simulink model "aero_guidance"  (R2019b)
settings: Solver=ode45  StartTime=0.0  StopTime=20  RelTol=1e-3  AbsTol=1e-6
PreLoadFcn:
  | aero_guid_dat
StopFcn:
  | aero_guid_plot
undefined symbols (not defined in the file): Beamwidth, Cm_el, Cm_q, Cz_el, d2r, d_ref, fin_max, fin_min, g, h_ini, K_r, Ks, l_acc, max_acc, max_gimbal, min_gimbal, pos_tgt, S_ref, theta_tgt, Thrust, tors, v_tgt, wgyro, wn_hom, x_ini
libraries: simulink_need_slupdate x11, aerospace x5, simulink x1
CloseFcn:
  | h=findobj('type','figure');if ~isempty(h);close(h);end
Description:
  | Dynamics of a missile engaging a target which is flying straight and level
settings Model: ExtModeTrigMode=oneshot  ExtModeArmWhenConnect=off  ExtModeAutoUpdateStatusClock=off  Creator=The MathWorks, Inc.  LastModifiedBy=Eduardo
settings SolverCC: AutoScaleAbsTol=off
settings DataIOCC: SaveFormat=Array  SaveOutput=off  ReturnWorkspaceOutputs=off  StateSaveName=xbase  OutputSaveName=ybase  SignalLoggingName=sigsOut
settings OptimizationCC: BlockReduction=off  ExpressionDepthLimit=2147483647  InitFltsAndDblsToZero=on  LifeSpan=inf
settings DebuggingCC: SaveWithParameterizedLinksMsg=none  SignalResolutionControl=TryResolveAllWithWarning  MultiTaskDSMMsg=warning  MultiTaskCondExecSysMsg=none  SigSpecEnsureSampleTimeMsg=none  FcnCallInpInsideContextMsg=warning  StateNameClashWarn=warning  SFUnexpectedBacktrackingDiag=warning  SFNoUnconditionalDefaultTransitionDiag=warning  SFExecutionAtInitializationDiag=none  ArithmeticOperatorsInVariantConditions=warning
settings HardwareCC: ProdBitPerPointer=32  ProdBitPerSizeT=32  ProdBitPerPtrDiffT=32  ProdLargestAtomicFloat=None  ProdIntDivRoundTo=Undefined  ProdEndianess=Unspecified  ProdWordSize=32  ProdHWDeviceType=32-bit Generic
settings ModelReferenceCC: PropagateSignalLabelsOutOfModel=off
settings SFSimCC: SimUseLocalCustomCode=off  SimParseCustomCode=off  CustomCodeUndefinedFunction=UseInterfaceOnly
settings RTWCC: RTWUseLocalCustomCode=off
settings CodeAppCC: StateflowObjectComments=on
settings GRTTargetCC: TargetFcnLib=ansi_tfl_tmw.mat  TargetLangStandard=C89/C90 (ANSI)  GeneratePreprocessorConditionals=Disable all  CombineOutputUpdateFcns=off  GRTInterface=on
settings ConfigComp: CovMetricSettings=d  CovHtmlReporting=on  CovSaveCumulativeToWorkspaceVar=on  CovSaveSingleToWorkspaceVar=on  CovExternalEMLEnable=off  CovSFcnEnable=off

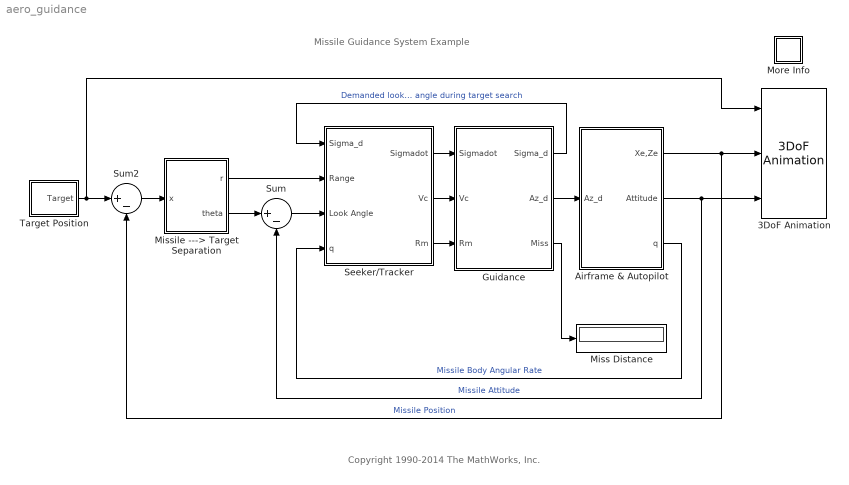
== system aero_guidance ==
  note: Copyright 1990-2014 The MathWorks, Inc.
  note: Missile Guidance System Example
  3DoF Animation : aerospace/Animation/3DoF Animation  u1=[0 5000 -2000 2000 -5050 -3050]  u2=0.03  u3=1.8  u5=Fly alongside  u6=[200 200 -50]  u7=20  u8=on
  Airframe & Autopilot : Subsystem
  Guidance : Subsystem
  Miss Distance : Display
  Missile ---> Target Separation : Subsystem  mask(Cart2Polar){}
      mask help:
      | Transformation from cartesian to polar coordinates.
      | [x, y] -> [r, theta]
      |
      | r = sqrt(x^2 + y^2);
      | theta = atan(y/x);
      mask Help: Unmask this block for more help.
      mask Display: plot(0,0,100,100,[24,20,15,20,20],[85,95,85,95,20],[80,20,95,85,95,85],[70,20,20,15,20,24],[56,56,55,52,50,46],[20,26,31,35,38,42])
  More Info : Subsystem
      settings: OpenFcn=showdemo(bdroot(gcb))
      mask Display: disp('?')
  Seeker/Tracker : Subsystem
  Sum : Sum  Inputs=|+-  SaturateOnIntegerOverflow=on  InputSameDT=on  OutDataTypeStr=Inherit: Same as first input
  Sum2 : Sum  Inputs=|+-  SaturateOnIntegerOverflow=on  InputSameDT=on  OutDataTypeStr=Inherit: Same as first input
  Target Position : Subsystem
  wires:
  Missile ---> Target Separation/2(theta) -> Sum/1
  Guidance/2(Az_d) -> Airframe & Autopilot/1(Az_d)
  Seeker/Tracker/2(Vc) -> Guidance/2(Vc)
  Seeker/Tracker/3(Rm) -> Guidance/3(Rm)
  Guidance/3(Miss) -> Miss Distance/1
  Seeker/Tracker/1(Sigmadot) -> Guidance/1(Sigmadot)
  Sum/1 -> Seeker/Tracker/3(Look Angle)
  Airframe & Autopilot/3(q) -> Seeker/Tracker/4(q)  "Missile Body Angular Rate"
  Guidance/1(Sigma_d) -> Seeker/Tracker/1(Sigma_d)  "Demanded look angle during target search"
  Missile ---> Target Separation/1(r) -> Seeker/Tracker/2(Range)
  Airframe & Autopilot/1(Xe,Ze) -> 3DoF Animation/2, Sum2/2  "Missile Position"
  Airframe & Autopilot/2(Attitude) -> 3DoF Animation/3, Sum/2  "Missile Attitude"
  Target Position/1(Target) -> Sum2/1, 3DoF Animation/1
  Sum2/1 -> Missile ---> Target Separation/1(x)

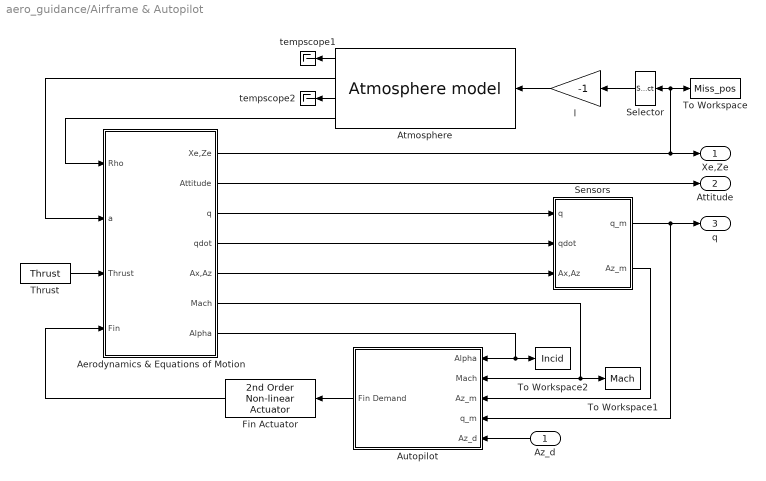
== system aero_guidance/Airframe & Autopilot ==
  Az_d : Inport
  Aerodynamics & Equations of Motion : Subsystem
  Atmosphere : aerospace/Atmosphere/Atmosphere model
  Autopilot : Subsystem
  Fin Actuator : aerospace/Actuators/2nd Order Non-linear Actuator  wn_fin=wn_fin  z_fin=z_fin  fin_max=fin_max  fin_min=fin_min  fin_maxrate=fin_maxrate  fin_act_0=fin_act_0
  Selector : Selector  InputPortWidth=2  IndexOptions=Index vector (dialog)  Indices=[2]  OutputSizes=1
  Sensors : Subsystem
  Thrust : Constant  Value=Thrust
  To Workspace : ToWorkspace  VariableName=Miss_pos  SaveFormat=Structure With Time  SampleTime=-1
  To Workspace1 : ToWorkspace  VariableName=Mach  SaveFormat=Structure With Time  SampleTime=-1
  To Workspace2 : ToWorkspace  VariableName=Incid  SaveFormat=Structure With Time  SampleTime=-1
  l : Gain  Gain=-1  SaturateOnIntegerOverflow=on  OutDataTypeStr=Inherit: Same as input  ParamDataTypeStr=Inherit: Same as input
  tempscope1 : Terminator
  tempscope2 : Terminator
  Xe,Ze : Outport  InitialOutput=0  VectorParamsAs1DForOutWhenUnconnected=off
  Attitude : Outport  Port=2  InitialOutput=0  VectorParamsAs1DForOutWhenUnconnected=off
  q : Outport  Port=3  InitialOutput=0  VectorParamsAs1DForOutWhenUnconnected=off
  wires:
  Aerodynamics & Equations of Motion/2(Attitude) -> Attitude/1
  Thrust/1 -> Aerodynamics & Equations of Motion/3(Thrust)
  Atmosphere/3 -> tempscope2/1
  Atmosphere/4 -> Aerodynamics & Equations of Motion/1(Rho)
  Atmosphere/1 -> tempscope1/1
  Atmosphere/2 -> Aerodynamics & Equations of Motion/2(a)
  Selector/1 -> l/1
  l/1 -> Atmosphere/1
  Aerodynamics & Equations of Motion/5(Ax,Az) -> Sensors/3(Ax,Az)
  Aerodynamics & Equations of Motion/4(qdot) -> Sensors/2(qdot)
  Aerodynamics & Equations of Motion/1(Xe,Ze) -> Xe,Ze/1, To Workspace/1, Selector/1
  Az_d/1 -> Autopilot/5(Az_d)
  Autopilot/1(Fin Demand) -> Fin Actuator/1
  Fin Actuator/1 -> Aerodynamics & Equations of Motion/4(Fin)
  Aerodynamics & Equations of Motion/7(Alpha) -> Autopilot/1(Alpha), To Workspace2/1
  Sensors/2(Az_m) -> Autopilot/3(Az_m)
  Aerodynamics & Equations of Motion/6(Mach) -> Autopilot/2(Mach), To Workspace1/1
  Sensors/1(q_m) -> Autopilot/4(q_m), q/1
  Aerodynamics & Equations of Motion/3(q) -> Sensors/1(q)

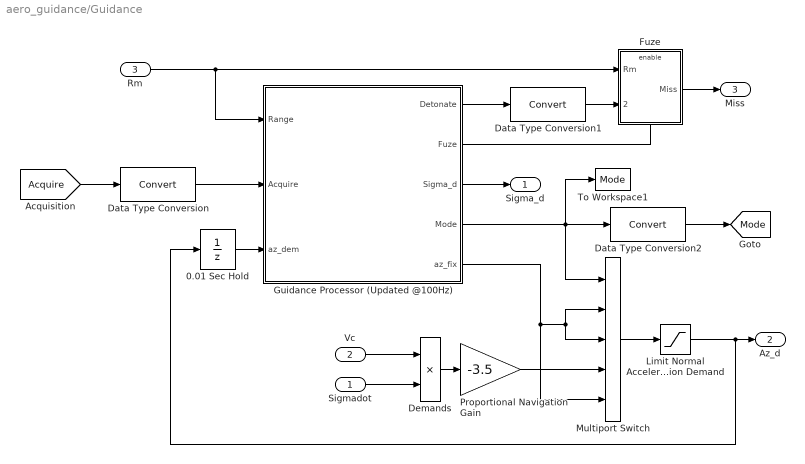
== system aero_guidance/Guidance ==
  Sigmadot : Inport
  Vc : Inport  Port=2
  Rm : Inport  Port=3
  0.01 Sec Hold : UnitDelay  SampleTime=0.01  HasFrameUpgradeWarning=on
  Data Type Conversion : DataTypeConversion
  Data Type Conversion1 : DataTypeConversion
  Data Type Conversion2 : DataTypeConversion
  Demands : Product  SaturateOnIntegerOverflow=on  InputSameDT=on  OutDataTypeStr=Inherit: Same as first input
  Fuze : Subsystem  TreatAsAtomicUnit=on
  Guidance Processor (Updated @100Hz) : Stateflow chart  TreatAsAtomicUnit=on
  "Limit Normal Acceleration Demand " : Saturate  UpperLimit=max_acc  LowerLimit=-max_acc
  Multiport Switch : MultiPortSwitch  Inputs=4  SaturateOnIntegerOverflow=on  InputSameDT=on
  Proportional Navigation Gain : Gain  Gain=-3.5  SaturateOnIntegerOverflow=on  OutDataTypeStr=Inherit: Same as input  ParamDataTypeStr=Inherit: Same as input
  To Workspace1 : ToWorkspace  VariableName=Mode  SaveFormat=Structure With Time
  Sigma_d : Outport  VectorParamsAs1DForOutWhenUnconnected=off
  Az_d : Outport  Port=2  VectorParamsAs1DForOutWhenUnconnected=off
  Miss : Outport  Port=3  VectorParamsAs1DForOutWhenUnconnected=off
  tag scope: Mode=global
  wires:
  Fuze/1("Miss ") -> Miss/1
  Guidance Processor (Updated @100Hz)/3(Sigma_d) -> Sigma_d/1
  [Acquire] -> Data Type Conversion/1
  Multiport Switch/1 -> "Limit Normal Acceleration Demand "/1
  Guidance Processor (Updated @100Hz)/1(Detonate) -> Data Type Conversion1/1
  "Limit Normal Acceleration Demand "/1 -> Az_d/1, 0.01 Sec Hold/1
  Guidance Processor (Updated @100Hz)/5(az_fix) -> Multiport Switch/2, Multiport Switch/3, Multiport Switch/5
  0.01 Sec Hold/1 -> Guidance Processor (Updated @100Hz)/3(az_dem)
  Sigmadot/1 -> Demands/2
  Proportional Navigation Gain/1 -> Multiport Switch/4
  Vc/1 -> Demands/1
  Demands/1 -> Proportional Navigation Gain/1
  Rm/1 -> Fuze/1(Rm), Guidance Processor (Updated @100Hz)/1(Range)
  Guidance Processor (Updated @100Hz)/2(Fuze) -> Fuze/Enable
  Guidance Processor (Updated @100Hz)/4(Mode) -> Data Type Conversion2/1, To Workspace1/1, Multiport Switch/1
  Data Type Conversion/1 -> Guidance Processor (Updated @100Hz)/2(Acquire)
  Data Type Conversion1/1 -> Fuze/2(Detonate)
  Data Type Conversion2/1 -> [Mode]

== system aero_guidance/Missile ---> Target Separation ==
  x : Inport
  Range : Fcn  Expr=hypot(u[1],u[2])
  Sightline Angle : Fcn  Expr=atan2(-u[2],u[1])
  r : Outport  InitialOutput=0  VectorParamsAs1DForOutWhenUnconnected=off
  theta : Outport  Port=2  InitialOutput=0  VectorParamsAs1DForOutWhenUnconnected=off
  wires:
  x/1 -> Sightline Angle/1, Range/1
  Range/1 -> r/1
  Sightline Angle/1 -> theta/1

== system aero_guidance/More Info ==

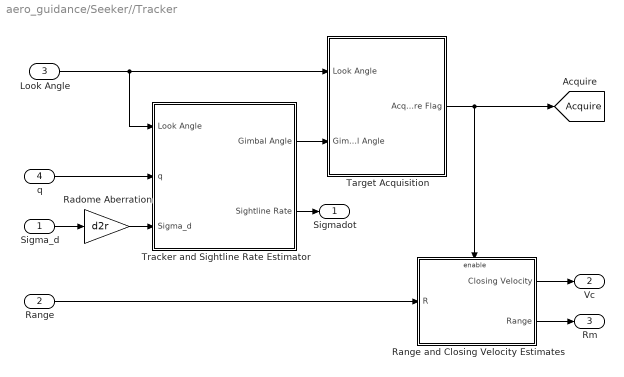
== system aero_guidance/Seeker//Tracker ==
  Sigma_d : Inport
  Range : Inport  Port=2
  Look Angle : Inport  Port=3
  q : Inport  Port=4
  Radome Aberration : Gain  Gain=d2r  SaturateOnIntegerOverflow=on  OutDataTypeStr=Inherit: Same as input  ParamDataTypeStr=Inherit: Same as input
  Range and Closing Velocity Estimates : Subsystem  TreatAsAtomicUnit=on
  Target Acquisition : Subsystem
  Tracker and Sightline Rate Estimator : Subsystem
  Sigmadot : Outport  VectorParamsAs1DForOutWhenUnconnected=off
  Vc : Outport  Port=2  VectorParamsAs1DForOutWhenUnconnected=off
  Rm : Outport  Port=3  VectorParamsAs1DForOutWhenUnconnected=off
  tag scope: Acquire=global
  wires:
  Tracker and Sightline Rate Estimator/2(Sightline Rate) -> Sigmadot/1
  Radome Aberration/1 -> Tracker and Sightline Rate Estimator/3(Sigma_d)
  Tracker and Sightline Rate Estimator/1("Gimbal Angle ") -> Target Acquisition/2(Gimbal Angle)
  Target Acquisition/1(Acquire Flag) -> [Acquire], Range and Closing Velocity Estimates/Enable
  q/1 -> Tracker and Sightline Rate Estimator/2(q)
  Look Angle/1 -> Target Acquisition/1(Look Angle), Tracker and Sightline Rate Estimator/1(Look Angle)
  Range/1 -> Range and Closing Velocity Estimates/1(R)
  Range and Closing Velocity Estimates/2(Range) -> Rm/1
  Range and Closing Velocity Estimates/1(Closing Velocity) -> Vc/1
  Sigma_d/1 -> Radome Aberration/1

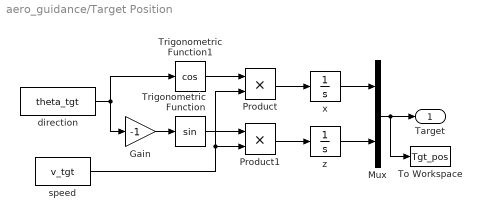
== system aero_guidance/Target Position ==
  Gain : Gain  Gain=-1  SaturateOnIntegerOverflow=on  OutDataTypeStr=Inherit: Same as input  ParamDataTypeStr=Inherit: Same as input
  Mux : Mux  Inputs=2
  Product : Product  SaturateOnIntegerOverflow=on  InputSameDT=on  OutDataTypeStr=Inherit: Same as first input
  Product1 : Product  SaturateOnIntegerOverflow=on  InputSameDT=on  OutDataTypeStr=Inherit: Same as first input
  To Workspace : ToWorkspace  VariableName=Tgt_pos  SaveFormat=Structure  SampleTime=-1
  Trigonometric Function : Trigonometry
  Trigonometric Function1 : Trigonometry  Operator=cos
  direction : Constant  Value=theta_tgt
  speed : Constant  Value=v_tgt
  x : Integrator  InitialCondition=pos_tgt(1)
  z : Integrator  InitialCondition=pos_tgt(2)
  Target : Outport  VectorParamsAs1DForOutWhenUnconnected=off
  wires:
  x/1 -> Mux/1
  z/1 -> Mux/2
  Product/1 -> x/1
  Product1/1 -> z/1
  speed/1 -> Product/2, Product1/2
  Trigonometric Function/1 -> Product1/1
  Trigonometric Function1/1 -> Product/1
  direction/1 -> Trigonometric Function1/1, Gain/1
  Gain/1 -> Trigonometric Function/1
  Mux/1 -> Target/1, To Workspace/1

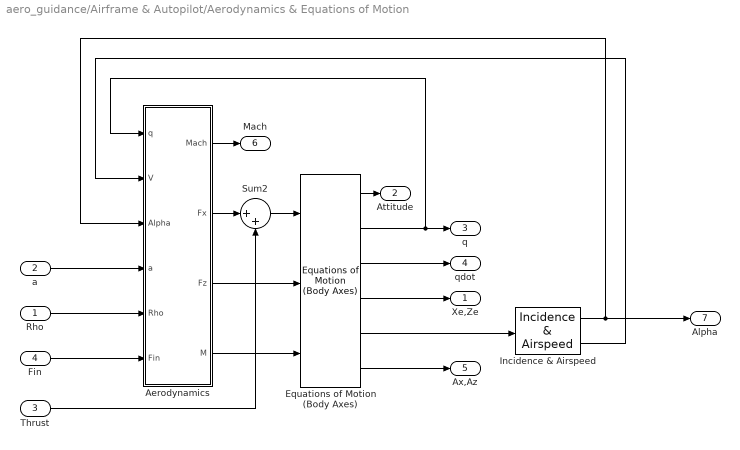
== system aero_guidance/Airframe & Autopilot/Aerodynamics & Equations of Motion ==
  Rho : Inport
  a : Inport  Port=2
  Thrust : Inport  Port=3
  Fin : Inport  Port=4
  " Equations of Motion (Body Axes)" : aerospace/3DoF Equations of Motion / Equations of Motion (Body Axes)  v_ini=v_ini  theta_ini=theta_ini  alpha_ini=alpha_ini  q_ini=q_ini  pos_ini=[x_ini -h_ini]  mass=mass  Iyy=Iyy  g=g
  Aerodynamics : Subsystem
  Incidence & Airspeed : aerospace/3DoF Equations of Motion /Incidence  & Airspeed
  Sum2 : Sum  Inputs=|++  SaturateOnIntegerOverflow=on  InputSameDT=on  OutDataTypeStr=Inherit: Same as first input
  Xe,Ze : Outport  InitialOutput=0  VectorParamsAs1DForOutWhenUnconnected=off
  Attitude : Outport  Port=2  InitialOutput=0  VectorParamsAs1DForOutWhenUnconnected=off
  q : Outport  Port=3  InitialOutput=0  VectorParamsAs1DForOutWhenUnconnected=off
  qdot : Outport  Port=4  InitialOutput=0  VectorParamsAs1DForOutWhenUnconnected=off
  Ax,Az : Outport  Port=5  InitialOutput=0  VectorParamsAs1DForOutWhenUnconnected=off
  Mach : Outport  Port=6  InitialOutput=0  VectorParamsAs1DForOutWhenUnconnected=off
  Alpha : Outport  Port=7  InitialOutput=0  VectorParamsAs1DForOutWhenUnconnected=off
  wires:
  Aerodynamics/1(" Mach") -> Mach/1
  Aerodynamics/4(" M") -> " Equations of Motion (Body Axes)"/3
  Sum2/1 -> " Equations of Motion (Body Axes)"/1
  Incidence & Airspeed/1 -> Aerodynamics/3(Alpha), Alpha/1
  Rho/1 -> Aerodynamics/5(Rho)
  a/1 -> Aerodynamics/4(a)
  Fin/1 -> Aerodynamics/6(Fin)
  Incidence & Airspeed/2 -> Aerodynamics/2(V)
  Aerodynamics/3(Fz) -> " Equations of Motion (Body Axes)"/2
  " Equations of Motion (Body Axes)"/2 -> q/1, Aerodynamics/1(q)
  " Equations of Motion (Body Axes)"/3 -> qdot/1
  " Equations of Motion (Body Axes)"/1 -> Attitude/1
  " Equations of Motion (Body Axes)"/4 -> Xe,Ze/1
  " Equations of Motion (Body Axes)"/6 -> Ax,Az/1
  " Equations of Motion (Body Axes)"/5 -> Incidence & Airspeed/1
  Aerodynamics/2(Fx) -> Sum2/1
  Thrust/1 -> Sum2/2

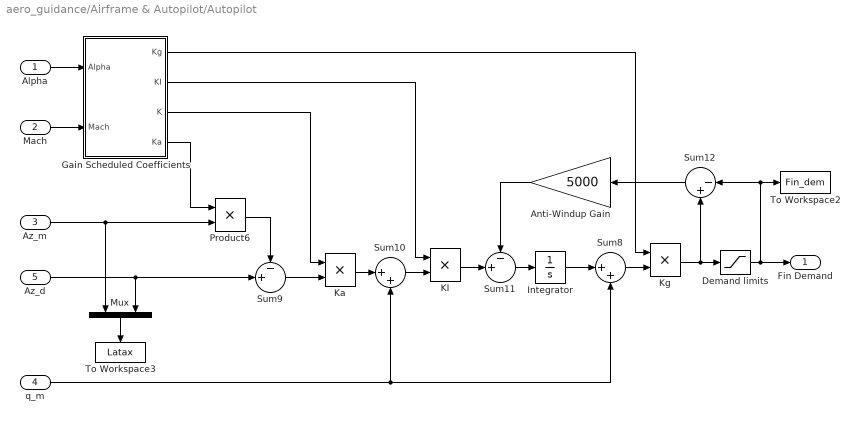
== system aero_guidance/Airframe & Autopilot/Autopilot ==
  Alpha : Inport
  Mach : Inport  Port=2
  Az_m : Inport  Port=3
  q_m : Inport  Port=4
  Az_d : Inport  Port=5
  Anti-Windup Gain : Gain  Gain=5000  SaturateOnIntegerOverflow=on  OutDataTypeStr=Inherit: Same as input  ParamDataTypeStr=Inherit: Same as input
  "Demand limits " : Saturate  UpperLimit=fin_max  LowerLimit=fin_min
  Gain Scheduled Coefficients : Subsystem
  Integrator : Integrator
  KI : Product  SaturateOnIntegerOverflow=on  InputSameDT=on  OutDataTypeStr=Inherit: Same as first input
  Ka : Product  SaturateOnIntegerOverflow=on  InputSameDT=on  OutDataTypeStr=Inherit: Same as first input
  Kg : Product  SaturateOnIntegerOverflow=on  InputSameDT=on  OutDataTypeStr=Inherit: Same as first input
  Mux : Mux  Inputs=2
  Product6 : Product  SaturateOnIntegerOverflow=on  InputSameDT=on  OutDataTypeStr=Inherit: Same as first input
  Sum10 : Sum  Inputs=|++  SaturateOnIntegerOverflow=on  InputSameDT=on  OutDataTypeStr=Inherit: Same as first input
  Sum11 : Sum  Inputs=-+|  SaturateOnIntegerOverflow=on  InputSameDT=on  OutDataTypeStr=Inherit: Same as first input
  Sum12 : Sum  Inputs=|-+  SaturateOnIntegerOverflow=on  InputSameDT=on  OutDataTypeStr=Inherit: Same as first input
  Sum8 : Sum  Inputs=|++  SaturateOnIntegerOverflow=on  InputSameDT=on  OutDataTypeStr=Inherit: Same as first input
  Sum9 : Sum  Inputs=-+|  SaturateOnIntegerOverflow=on  InputSameDT=on  OutDataTypeStr=Inherit: Same as first input
  To Workspace2 : ToWorkspace  VariableName=Fin_dem  SaveFormat=Structure With Time  SampleTime=-1
  To Workspace3 : ToWorkspace  VariableName=Latax  SaveFormat=Structure With Time  SampleTime=-1
  Fin Demand : Outport  InitialOutput=0  VectorParamsAs1DForOutWhenUnconnected=off
  wires:
  Mach/1 -> Gain Scheduled Coefficients/2(Mach)
  Alpha/1 -> Gain Scheduled Coefficients/1(Alpha)
  Kg/1 -> Sum12/2, "Demand limits "/1
  Gain Scheduled Coefficients/1("Kg ") -> Kg/1
  Gain Scheduled Coefficients/3("K ") -> Ka/1
  Gain Scheduled Coefficients/2("KI ") -> KI/1
  Anti-Windup Gain/1 -> Sum11/1
  Sum8/1 -> Kg/2
  Integrator/1 -> Sum8/1
  Sum11/1 -> Integrator/1
  Product6/1 -> Sum9/1
  Sum9/1 -> Ka/2
  Ka/1 -> Sum10/1
  Sum10/1 -> KI/2
  KI/1 -> Sum11/2
  Sum12/1 -> Anti-Windup Gain/1
  Az_d/1 -> Mux/2, Sum9/2
  Mux/1 -> To Workspace3/1
  q_m/1 -> Sum10/2, Sum8/2
  "Demand limits "/1 -> Fin Demand/1, Sum12/1, To Workspace2/1
  Az_m/1 -> Mux/1, Product6/2
  Gain Scheduled Coefficients/4("Ka ") -> Product6/1

== system aero_guidance/Airframe & Autopilot/Sensors ==
  q : Inport
  qdot : Inport  Port=2
  Ax,Az : Inport  Port=3
  Selector : Selector  InputPortWidth=2  IndexOptions=Index vector (dialog)  Indices=[2]  OutputSizes=1
  Sum : Sum  Inputs=-+|  SaturateOnIntegerOverflow=on  InputSameDT=on  OutDataTypeStr=Inherit: Same as first input
  l : Gain  Gain=l_acc  SaturateOnIntegerOverflow=on  OutDataTypeStr=Inherit: Same as input  ParamDataTypeStr=Inherit: Same as input
  q_m : Outport  InitialOutput=0  VectorParamsAs1DForOutWhenUnconnected=off
  Az_m : Outport  Port=2  InitialOutput=0  VectorParamsAs1DForOutWhenUnconnected=off
  wires:
  Selector/1 -> Sum/2
  Ax,Az/1 -> Selector/1
  q/1 -> q_m/1  "Rate Gyro"
  l/1 -> Sum/1
  Sum/1 -> Az_m/1  "Accelerometer"
  qdot/1 -> l/1

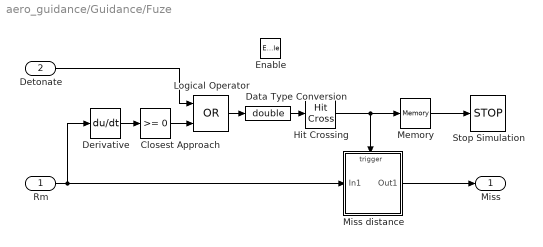
== system aero_guidance/Guidance/Fuze ==
  Rm : Inport
  Detonate : Inport  Port=2
  Enable : EnablePort
  Closest Approach : simulink/Logic and Bit Operations/Compare To Zero  relop=>=  OutDataTypeStr=boolean
  Data Type Conversion : DataTypeConversion  OutDataTypeStr=double
  Derivative : Derivative
  Hit Crossing : HitCross  HitCrossingDirection=rising
  Logical Operator : Logic  Operator=OR  IconShape=distinctive  OutDataTypeStr=boolean
  Memory : Memory
  Miss distance : Subsystem  TreatAsAtomicUnit=on
  Stop Simulation : Stop
  "Miss " : Outport  VectorParamsAs1DForOutWhenUnconnected=off
  wires:
  Derivative/1 -> Closest Approach/1
  Detonate/1 -> Logical Operator/1
  Rm/1 -> Miss distance/1(In1), Derivative/1
  Closest Approach/1 -> Logical Operator/2
  Memory/1 -> Stop Simulation/1
  Miss distance/1(Out1) -> "Miss "/1
  Hit Crossing/1 -> Miss distance/Trigger, Memory/1
  Data Type Conversion/1 -> Hit Crossing/1
  Logical Operator/1 -> Data Type Conversion/1

== system aero_guidance/Seeker//Tracker/Range and Closing Velocity Estimates ==
  R : Inport
  Enable : EnablePort  StatesWhenEnabling=reset
  Bandwidth of Estimator : Gain  Gain=wn_hom  SaturateOnIntegerOverflow=on  OutDataTypeStr=Inherit: Same as input  ParamDataTypeStr=Inherit: Same as input
  Initialized at acquisition : Integrator  InitialConditionSource=external
  Rdot ---> Vc : Gain  Gain=-1  SaturateOnIntegerOverflow=on  OutDataTypeStr=Inherit: Same as input  ParamDataTypeStr=Inherit: Same as input
  Sum : Sum  Inputs=|+-  SaturateOnIntegerOverflow=on  InputSameDT=on  OutDataTypeStr=Inherit: Same as first input
  Closing Velocity : Outport  InitialOutput=0  VectorParamsAs1DForOutWhenUnconnected=off
  Range : Outport  Port=2  InitialOutput=0  VectorParamsAs1DForOutWhenUnconnected=off
  wires:
  R/1 -> Range/1, Initialized at acquisition/2, Sum/1
  Sum/1 -> Bandwidth of Estimator/1
  Initialized at acquisition/1 -> Sum/2
  Bandwidth of Estimator/1 -> Rdot ---> Vc/1, Initialized at acquisition/1
  Rdot ---> Vc/1 -> Closing Velocity/1

== system aero_guidance/Seeker//Tracker/Target Acquisition ==
  Look Angle : Inport
  Gimbal Angle : Inport  Port=2
  Abs : Abs  SaturateOnIntegerOverflow=on
  Beamwidth : Constant  Value=Beamwidth/2
  Mux : Mux  Inputs=2
  Relational Operator : RelationalOperator  Operator=<  OutDataTypeStr=boolean  RndMeth=Nearest  InputSameDT=on
  Sum : Sum  Inputs=+-  SaturateOnIntegerOverflow=on  InputSameDT=on  OutDataTypeStr=Inherit: Same as first input
  To Workspace2 : ToWorkspace  VariableName=Gimbal  SaveFormat=Structure With Time  SampleTime=-1
  Acquire Flag : Outport  VectorParamsAs1DForOutWhenUnconnected=off
  wires:
  Look Angle/1 -> Sum/2, Mux/2
  Gimbal Angle/1 -> Sum/1, Mux/1
  Mux/1 -> To Workspace2/1
  Sum/1 -> Abs/1
  Beamwidth/1 -> Relational Operator/2
  Relational Operator/1 -> Acquire Flag/1
  Abs/1 -> Relational Operator/1

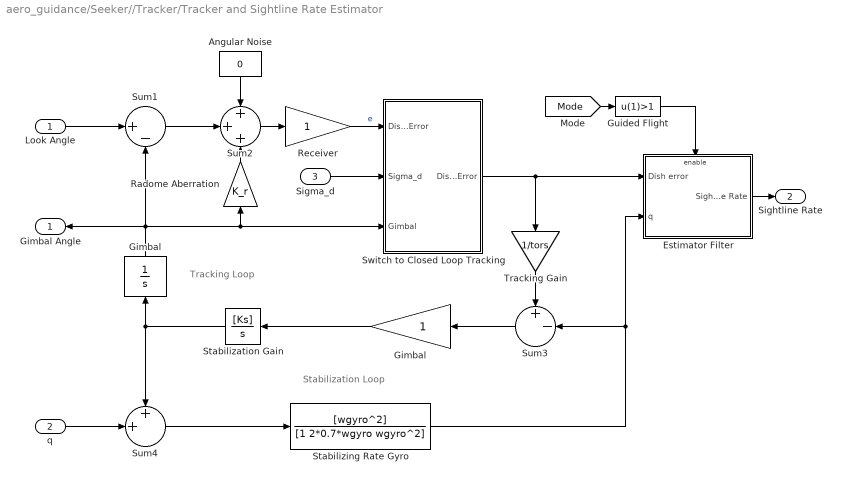
== system aero_guidance/Seeker//Tracker/Tracker and Sightline Rate Estimator ==
  note: Stabilization Loop
  note: Tracking Loop
  Look Angle : Inport
  q : Inport  Port=2
  Sigma_d : Inport  Port=3
  Angular Noise : Constant  Value=0
  Estimator Filter : Subsystem  TreatAsAtomicUnit=on
  Gimbal : Gain  SaturateOnIntegerOverflow=on  OutDataTypeStr=Inherit: Same as input  ParamDataTypeStr=Inherit: Same as input
  "Gimbal " : Integrator  LimitOutput=on  UpperSaturationLimit=max_gimbal  LowerSaturationLimit=min_gimbal
  Guided Flight : Fcn  Expr=u(1)>1
  Radome Aberration : Gain  Gain=K_r  SaturateOnIntegerOverflow=on  OutDataTypeStr=Inherit: Same as input  ParamDataTypeStr=Inherit: Same as input
  Receiver : Gain  SaturateOnIntegerOverflow=on  OutDataTypeStr=Inherit: Same as input  ParamDataTypeStr=Inherit: Same as input
  Stabilization Gain : TransferFcn  Numerator=[Ks]  Denominator=[1 0]
  Stabilizing Rate Gyro : TransferFcn  Numerator=[wgyro^2]  Denominator=[1 2*0.7*wgyro wgyro^2]
  Sum1 : Sum  Inputs=|+-  SaturateOnIntegerOverflow=on  InputSameDT=on  OutDataTypeStr=Inherit: Same as first input
  Sum2 : Sum  Inputs=+++  SaturateOnIntegerOverflow=on  InputSameDT=on  OutDataTypeStr=Inherit: Same as first input
  Sum3 : Sum  Inputs=+-|  SaturateOnIntegerOverflow=on  InputSameDT=on  OutDataTypeStr=Inherit: Same as first input
  Sum4 : Sum  Inputs=++|  SaturateOnIntegerOverflow=on  InputSameDT=on  OutDataTypeStr=Inherit: Same as first input
  Switch to Closed Loop Tracking : Subsystem
  Tracking Gain : Gain  Gain=1/tors  SaturateOnIntegerOverflow=on  OutDataTypeStr=Inherit: Same as input  ParamDataTypeStr=Inherit: Same as input
  "Gimbal Angle " : Outport  VectorParamsAs1DForOutWhenUnconnected=off
  Sightline Rate : Outport  Port=2  VectorParamsAs1DForOutWhenUnconnected=off
  wires:
  "Gimbal "/1 -> Sum1/2, Radome Aberration/1, Switch to Closed Loop Tracking/3(Gimbal), "Gimbal Angle "/1
  Stabilization Gain/1 -> "Gimbal "/1, Sum4/1
  Gimbal/1 -> Stabilization Gain/1
  Look Angle/1 -> Sum1/1
  Sum2/1 -> Receiver/1
  Receiver/1 -> Switch to Closed Loop Tracking/1(Dish Error)  "e"
  Sigma_d/1 -> Switch to Closed Loop Tracking/2(Sigma_d)
  Estimator Filter/1(Sightline Rate) -> Sightline Rate/1
  Radome Aberration/1 -> Sum2/3
  Sum1/1 -> Sum2/2
  Angular Noise/1 -> Sum2/1
  Sum4/1 -> Stabilizing Rate Gyro/1
  q/1 -> Sum4/2
  Stabilizing Rate Gyro/1 -> Sum3/2, Estimator Filter/2(q)
  Sum3/1 -> Gimbal/1
  Tracking Gain/1 -> Sum3/1
  Switch to Closed Loop Tracking/1("Dish Error ") -> Tracking Gain/1, Estimator Filter/1(Dish error)
  Guided Flight/1 -> Estimator Filter/Enable
  [Mode] -> Guided Flight/1

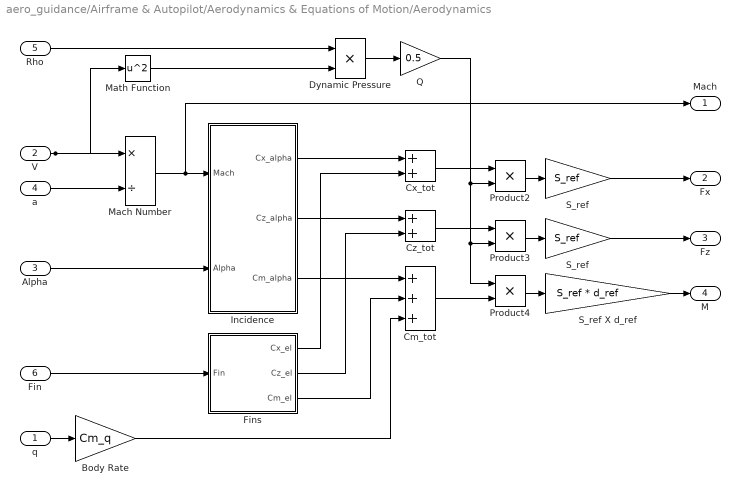
== system aero_guidance/Airframe & Autopilot/Aerodynamics & Equations of Motion/Aerodynamics ==
  q : Inport
  V : Inport  Port=2
  Alpha : Inport  Port=3
  a : Inport  Port=4
  Rho : Inport  Port=5
  Fin : Inport  Port=6
  Body Rate : Gain  Gain=Cm_q  SaturateOnIntegerOverflow=on  OutDataTypeStr=Inherit: Same as input  ParamDataTypeStr=Inherit: Same as input
  Cm_tot : Sum  Inputs=+++  SaturateOnIntegerOverflow=on  InputSameDT=on  OutDataTypeStr=Inherit: Same as first input
  Cx_tot : Sum  SaturateOnIntegerOverflow=on  InputSameDT=on  OutDataTypeStr=Inherit: Same as first input
  Cz_tot : Sum  SaturateOnIntegerOverflow=on  InputSameDT=on  OutDataTypeStr=Inherit: Same as first input
  Dynamic Pressure : Product  SaturateOnIntegerOverflow=on  InputSameDT=on  OutDataTypeStr=Inherit: Same as first input
  Fins : Subsystem
  Incidence : Subsystem
  Mach Number : Product  Inputs=*/  SaturateOnIntegerOverflow=on  InputSameDT=on  OutDataTypeStr=Inherit: Same as first input
  Math Function : Math  Operator=square  SaturateOnIntegerOverflow=on
  Product2 : Product  SaturateOnIntegerOverflow=on  InputSameDT=on  OutDataTypeStr=Inherit: Same as first input
  Product3 : Product  SaturateOnIntegerOverflow=on  InputSameDT=on  OutDataTypeStr=Inherit: Same as first input
  Product4 : Product  SaturateOnIntegerOverflow=on  InputSameDT=on  OutDataTypeStr=Inherit: Same as first input
  Q : Gain  Gain=0.5  SaturateOnIntegerOverflow=on  OutDataTypeStr=Inherit: Same as input  ParamDataTypeStr=Inherit: Same as input
  S_ref : Gain  Gain=S_ref  SaturateOnIntegerOverflow=on  OutDataTypeStr=Inherit: Same as input  ParamDataTypeStr=Inherit: Same as input
  "S_ref " : Gain  Gain=S_ref  SaturateOnIntegerOverflow=on  OutDataTypeStr=Inherit: Same as input  ParamDataTypeStr=Inherit: Same as input
  S_ref X d_ref : Gain  Gain=S_ref * d_ref  SaturateOnIntegerOverflow=on  OutDataTypeStr=Inherit: Same as input  ParamDataTypeStr=Inherit: Same as input
  " Mach" : Outport  InitialOutput=0  VectorParamsAs1DForOutWhenUnconnected=off
  Fx : Outport  Port=2  InitialOutput=[0]  VectorParamsAs1DForOutWhenUnconnected=off
  Fz : Outport  Port=3  InitialOutput=0  VectorParamsAs1DForOutWhenUnconnected=off
  " M" : Outport  Port=4  InitialOutput=0  VectorParamsAs1DForOutWhenUnconnected=off
  wires:
  Math Function/1 -> Dynamic Pressure/2
  Rho/1 -> Dynamic Pressure/1
  Dynamic Pressure/1 -> Q/1
  Q/1 -> Product2/2, Product3/2, Product4/1
  V/1 -> Math Function/1, Mach Number/1
  Incidence/1(Cx_alpha) -> Cx_tot/1
  Fins/1(Cx_el) -> Cx_tot/2
  Incidence/2(Cz_alpha) -> Cz_tot/1
  Fins/2(Cz_el) -> Cz_tot/2
  Incidence/3(Cm_alpha) -> Cm_tot/1
  Fins/3(Cm_el) -> Cm_tot/2
  Body Rate/1 -> Cm_tot/3
  a/1 -> Mach Number/2
  Alpha/1 -> Incidence/2(Alpha)
  Cx_tot/1 -> Product2/1
  Cz_tot/1 -> Product3/1
  Product2/1 -> S_ref/1
  S_ref/1 -> Fx/1
  Product3/1 -> "S_ref "/1
  "S_ref "/1 -> Fz/1
  Fin/1 -> Fins/1(Fin)
  S_ref X d_ref/1 -> " M"/1
  Product4/1 -> S_ref X d_ref/1
  Cm_tot/1 -> Product4/2
  q/1 -> Body Rate/1
  Mach Number/1 -> " Mach"/1, Incidence/1(Mach)

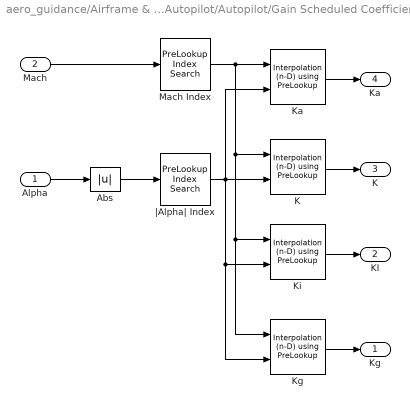
== system aero_guidance/Airframe & Autopilot/Autopilot/Gain Scheduled Coefficients ==
  Alpha : Inport
  Mach : Inport  Port=2
  Abs : Abs  SaturateOnIntegerOverflow=on
  K : simulink_need_slupdate/Interpolation (n-D) using PreLookup  numDimsPopupSelect=2  explicitNumDims=2  table=K  interpMethod=Linear  extrapMethod=Linear  rangeErrorMode=None  NumSelectionDims=0
      settings: SourceProductName=Simulink  SourceProductBaseCode=SL
  Ka : simulink_need_slupdate/Interpolation (n-D) using PreLookup  numDimsPopupSelect=2  explicitNumDims=2  table=Ka  interpMethod=Linear  extrapMethod=Linear  rangeErrorMode=None  NumSelectionDims=0
      settings: SourceProductName=Simulink  SourceProductBaseCode=SL
  Kg : simulink_need_slupdate/Interpolation (n-D) using PreLookup  numDimsPopupSelect=2  explicitNumDims=2  table=Kg  interpMethod=Linear  extrapMethod=Linear  rangeErrorMode=None  NumSelectionDims=0
      settings: SourceProductName=Simulink  SourceProductBaseCode=SL
  Ki : simulink_need_slupdate/Interpolation (n-D) using PreLookup  numDimsPopupSelect=2  explicitNumDims=2  table=Ki  interpMethod=Linear  extrapMethod=Linear  rangeErrorMode=None  NumSelectionDims=0
      settings: SourceProductName=Simulink  SourceProductBaseCode=SL
  Mach Index : simulink_need_slupdate/PreLookup Index Search  bpData=M_sch  searchMode=Binary Search  cacheBpFlag=on  outputFlag=off  IndexDataType=uint32  extrapMode=Linear Extrapolation  rangeErrorMode=None
      settings: SourceProductName=Simulink  SourceProductBaseCode=SL
  |Alpha| Index : simulink_need_slupdate/PreLookup Index Search  bpData=alpha_sch  searchMode=Binary Search  cacheBpFlag=on  outputFlag=off  IndexDataType=uint32  extrapMode=Linear Extrapolation  rangeErrorMode=None
      settings: SourceProductName=Simulink  SourceProductBaseCode=SL
  "Kg " : Outport  InitialOutput=0  VectorParamsAs1DForOutWhenUnconnected=off
  "KI " : Outport  Port=2  InitialOutput=0  VectorParamsAs1DForOutWhenUnconnected=off
  "K " : Outport  Port=3  InitialOutput=0  VectorParamsAs1DForOutWhenUnconnected=off
  "Ka " : Outport  Port=4  InitialOutput=0  VectorParamsAs1DForOutWhenUnconnected=off
  wires:
  Alpha/1 -> Abs/1
  Mach Index/1 -> Ka/1, K/1, Ki/1, Kg/1
  |Alpha| Index/1 -> Ka/2, K/2, Ki/2, Kg/2
  Ka/1 -> "Ka "/1
  K/1 -> "K "/1
  Ki/1 -> "KI "/1
  Kg/1 -> "Kg "/1
  Abs/1 -> |Alpha| Index/1
  Mach/1 -> Mach Index/1

== system aero_guidance/Guidance/Fuze/Miss distance ==
  In1 : Inport
  Trigger : TriggerPort  VariantControl=(inherit)
  Out1 : Outport  VectorParamsAs1DForOutWhenUnconnected=off
  wires:
  In1/1 -> Out1/1

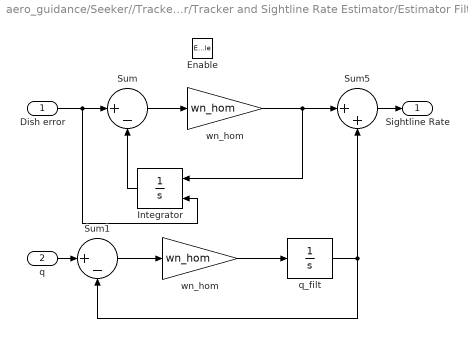
== system aero_guidance/Seeker//Tracker/Tracker and Sightline Rate Estimator/Estimator Filter ==
  Dish error : Inport
  q : Inport  Port=2
  Enable : EnablePort  StatesWhenEnabling=reset
  Integrator : Integrator  InitialConditionSource=external
  Sum : Sum  Inputs=|+-  SaturateOnIntegerOverflow=on  InputSameDT=on  OutDataTypeStr=Inherit: Same as first input
  Sum1 : Sum  Inputs=|+-  SaturateOnIntegerOverflow=on  InputSameDT=on  OutDataTypeStr=Inherit: Same as first input
  Sum5 : Sum  Inputs=|++  SaturateOnIntegerOverflow=on  InputSameDT=on  OutDataTypeStr=Inherit: Same as first input
  q_filt : Integrator
  wn_hom : Gain  Gain=wn_hom  SaturateOnIntegerOverflow=on  OutDataTypeStr=Inherit: Same as input  ParamDataTypeStr=Inherit: Same as input
  "wn_hom  " : Gain  Gain=wn_hom  SaturateOnIntegerOverflow=on  OutDataTypeStr=Inherit: Same as input  ParamDataTypeStr=Inherit: Same as input
  Sightline Rate : Outport  InitialOutput=0  VectorParamsAs1DForOutWhenUnconnected=off
  wires:
  Dish error/1 -> Sum/1, Integrator/2
  Sum/1 -> wn_hom/1
  Integrator/1 -> Sum/2
  Sum5/1 -> Sightline Rate/1
  wn_hom/1 -> Integrator/1, Sum5/1
  q/1 -> Sum1/1
  Sum1/1 -> "wn_hom  "/1
  "wn_hom  "/1 -> q_filt/1
  q_filt/1 -> Sum5/2, Sum1/2

== system aero_guidance/Seeker//Tracker/Tracker and Sightline Rate Estimator/Switch to Closed Loop Tracking ==
  Dish Error : Inport
  Sigma_d : Inport  Port=2
  Gimbal : Inport  Port=3
  Guided Flight : Fcn  Expr=u(1)>1
  Sum5 : Sum  Inputs=-+  SaturateOnIntegerOverflow=on  InputSameDT=on  OutDataTypeStr=Inherit: Same as first input
  Switch2 : Switch  Threshold=0.5  SaturateOnIntegerOverflow=on  InputSameDT=on
  "Dish Error " : Outport  VectorParamsAs1DForOutWhenUnconnected=off
  wires:
  [Mode] -> Guided Flight/1
  Guided Flight/1 -> Switch2/2
  Sum5/1 -> Switch2/3
  Dish Error/1 -> Switch2/1
  Switch2/1 -> "Dish Error "/1
  Sigma_d/1 -> Sum5/2
  Gimbal/1 -> Sum5/1

== system aero_guidance/Airframe & Autopilot/Aerodynamics & Equations of Motion/Aerodynamics/Fins ==
  Fin : Inport
  Cm : Gain  Gain=Cm_el  SaturateOnIntegerOverflow=on  OutDataTypeStr=Inherit: Same as input  ParamDataTypeStr=Inherit: Same as input
  Cx : Gain  Gain=0  SaturateOnIntegerOverflow=on  OutDataTypeStr=Inherit: Same as input  ParamDataTypeStr=Inherit: Same as input
  Cz : Gain  Gain=Cz_el  SaturateOnIntegerOverflow=on  OutDataTypeStr=Inherit: Same as input  ParamDataTypeStr=Inherit: Same as input
  Cx_el : Outport  InitialOutput=0  VectorParamsAs1DForOutWhenUnconnected=off
  Cz_el : Outport  Port=2  InitialOutput=0  VectorParamsAs1DForOutWhenUnconnected=off
  Cm_el : Outport  Port=3  InitialOutput=0  VectorParamsAs1DForOutWhenUnconnected=off
  wires:
  Fin/1 -> Cx/1, Cm/1, Cz/1
  Cx/1 -> Cx_el/1
  Cm/1 -> Cm_el/1
  Cz/1 -> Cz_el/1

== system aero_guidance/Airframe & Autopilot/Aerodynamics & Equations of Motion/Aerodynamics/Incidence ==
  Mach : Inport
  Alpha : Inport  Port=2
  Alpha Index : simulink_need_slupdate/PreLookup Index Search  bpData=alpha_vec  searchMode=Binary Search  cacheBpFlag=on  outputFlag=off  IndexDataType=uint32  extrapMode=Linear Extrapolation  rangeErrorMode=None
      settings: SourceProductName=Simulink  SourceProductBaseCode=SL
  Cm : simulink_need_slupdate/Interpolation (n-D) using PreLookup  numDimsPopupSelect=2  explicitNumDims=2  table=Cm_alpha  interpMethod=Linear  extrapMethod=Linear  rangeErrorMode=None  NumSelectionDims=0
      settings: SourceProductName=Simulink  SourceProductBaseCode=SL
  Cx : simulink_need_slupdate/Interpolation (n-D) using PreLookup  numDimsPopupSelect=2  explicitNumDims=2  table=Cx_alpha  interpMethod=Linear  extrapMethod=Linear  rangeErrorMode=None  NumSelectionDims=0
      settings: SourceProductName=Simulink  SourceProductBaseCode=SL
  Cz : simulink_need_slupdate/Interpolation (n-D) using PreLookup  numDimsPopupSelect=2  explicitNumDims=2  table=Cz_alpha  interpMethod=Linear  extrapMethod=Linear  rangeErrorMode=None  NumSelectionDims=0
      settings: SourceProductName=Simulink  SourceProductBaseCode=SL
  Mach Index : simulink_need_slupdate/PreLookup Index Search  bpData=Mach_vec  searchMode=Binary Search  cacheBpFlag=on  outputFlag=off  IndexDataType=uint32  extrapMode=Linear Extrapolation  rangeErrorMode=None
      settings: SourceProductName=Simulink  SourceProductBaseCode=SL
  Cx_alpha : Outport  InitialOutput=0  VectorParamsAs1DForOutWhenUnconnected=off
  Cz_alpha : Outport  Port=2  InitialOutput=0  VectorParamsAs1DForOutWhenUnconnected=off
  Cm_alpha : Outport  Port=3  InitialOutput=0  VectorParamsAs1DForOutWhenUnconnected=off
  wires:
  Alpha Index/1 -> Cx/1, Cz/1, Cm/1
  Mach Index/1 -> Cx/2, Cz/2, Cm/2
  Cx/1 -> Cx_alpha/1
  Cz/1 -> Cz_alpha/1
  Cm/1 -> Cm_alpha/1
  Alpha/1 -> Alpha Index/1
  Mach/1 -> Mach Index/1

== stateflow chart aero_guidance/Guidance/Guidance Processor (Updated @100Hz) ==
  settings: updateMethod=DISCRETE  sampleTime=0.01
  state Guidance [parallel]
    settings: executionOrder=1
    state Target_Search
      en: Mode=1;Sigma_d=0;incr=-100;Acquire_time=t;
      du: Sigma_d=Sigma_d+0.01*incr;
      Target_Search -> Target_Search [order 1] : [Sigma_d>30||Sigma_d<-30]  / incr=-incr;
    state Target_Lock
      en:Mode=2;Acquire_time=t;
    state Abort
      en:Detonate=1;
    state Radar_Guided
      en:Mode=3;
      ex:az_fix=az_dem;
    state Blind_Range
      en:Mode=4;
    (default) -> Target_Search : {az_fix=-9.81;}
    Radar_Guided -> Target_Search [order 1] : [Acquire==0]
    Target_Search -> Abort [order 2] : [t-Acquire_time>7]
        | / send(Timeout, Fuze);
    Target_Search -> Target_Lock [order 1] : [Acquire==1]
    Target_Lock -> Radar_Guided : [t-Acquire_time>0.2]
    Radar_Guided -> Blind_Range [order 2] : [Range<200]
  state Fuze [parallel]
    settings: executionOrder=2
    state Armed
      en:Fuze=1;
    state Inert
      en:Fuze = 0;
    Inert -> Armed [order 2] : [in(Guidance.Radar_Guided)&&Range<1000]
    (default) -> Inert
    Inert -> Armed [order 1] : Timeout
    Armed -> Inert : enter(Guidance.Target_Search)
  data: Range input double; Detonate output boolean; Fuze output boolean; Sigma_d output double; Mode output uint8; Acquire input boolean; Acquire_time local double; incr local double; az_dem input double; az_fix output double =-9.81
  data Sigma_d settings: description=Demanded Seeker Look Angle
  data Acquire settings: description=Seeker Acquisition Flag
  data incr settings: description=Seeker Search Rate
  events: Timeout local EITHER_EDGE_EVENT
